simulink model "twoFingerTest2015a"  (R2015a)
settings: Solver=ode45  StartTime=0.0  StopTime=1.0  RelTol=1e-3
settings Model: CovModelRefEnable=off  Creator=Ricardo  LastModifiedBy=Ricardo
settings DataIOCC: SaveFormat=Dataset
settings HardwareCC: ProdBitPerPointer=64  ProdLargestAtomicFloat=Float  ProdIntDivRoundTo=Zero  ProdEndianess=LittleEndian  ProdHWDeviceType=Specified
settings GRTTargetCC: GeneratePreprocessorConditionals=Use local settings

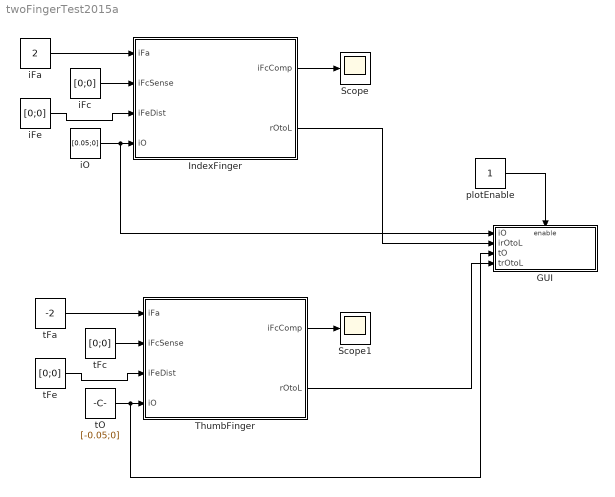
== system twoFingerTest2015a ==
  GUI : Subsystem  TreatAsAtomicUnit=on
  IndexFinger : Subsystem
  Scope : Scope
      settings: TimeRange=auto  MaxDataPoints=5000  SaveToWorkspace=off  SaveName=ScopeData  YMin=-0.27034  YMax=0.08548  SampleTime=-1
  Scope1 : Scope
      settings: TimeRange=auto  MaxDataPoints=5000  SaveToWorkspace=off  YMin=-0.03724  YMax=0.26498  SampleTime=-1
  ThumbFinger : Subsystem
  iFa : Constant  Value=2
  iFc : Constant  Value=[0;0]
  iFe : Constant  Value=[0;0]
  iO : Constant  Value=[0.05;0]
  plotEnable : Constant
  tFa : Constant  Value=-2
  tFc : Constant  Value=[0;0]
  tFe : Constant  Value=[0;0]
  tO : Constant  Value=[-0.05;0]
  wires:
  plotEnable/1 -> GUI/Enable
  IndexFinger/1(iFcComp) -> Scope/1
  iFc/1 -> IndexFinger/2(iFcSense)
  iFe/1 -> IndexFinger/3(iFeDist)
  iO/1 -> GUI/1(iO), IndexFinger/4(iO)
  iFa/1 -> IndexFinger/1(iFa)
  IndexFinger/2(rOtoL) -> GUI/2(irOtoL)
  tFe/1 -> ThumbFinger/3(iFeDist)
  tFa/1 -> ThumbFinger/1(iFa)
  tFc/1 -> ThumbFinger/2(iFcSense)
  tO/1 -> GUI/3(tO), ThumbFinger/4(iO)
  ThumbFinger/1(iFcComp) -> Scope1/1
  ThumbFinger/2(rOtoL) -> GUI/4(trOtoL)

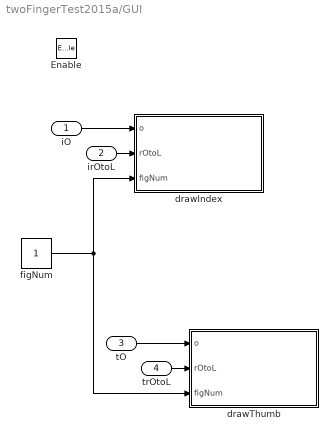
== system twoFingerTest2015a/GUI ==
  iO : Inport
  irOtoL : Inport  Port=2
  tO : Inport  Port=3
  trOtoL : Inport  Port=4
  Enable : EnablePort
  drawIndex : MATLAB Function  TreatAsAtomicUnit=on
      settings: PermitHierarchicalResolution=ParametersOnly
  drawThumb : MATLAB Function  TreatAsAtomicUnit=on
      settings: PermitHierarchicalResolution=ParametersOnly
  figNum : Constant
  wires:
  figNum/1 -> drawThumb/3(figNum), drawIndex/3(figNum)
  tO/1 -> drawThumb/1(o)
  trOtoL/1 -> drawThumb/2(rOtoL)
  irOtoL/1 -> drawIndex/2(rOtoL)
  iO/1 -> drawIndex/1(o)

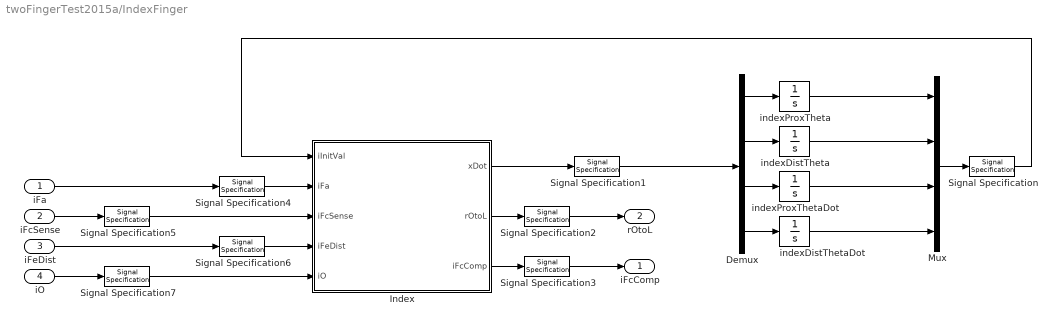
== system twoFingerTest2015a/IndexFinger ==
  iFa : Inport
  iFcSense : Inport  Port=2
  iFeDist : Inport  Port=3
  iO : Inport  Port=4
  Demux : Demux
  Index : MATLAB Function  TreatAsAtomicUnit=on
      settings: PermitHierarchicalResolution=ParametersOnly
  Mux : Mux
  Signal Specification : SignalSpecification  Dimensions=4
  Signal Specification1 : SignalSpecification  Dimensions=4
  Signal Specification2 : SignalSpecification  Dimensions=[2 2]
  Signal Specification{3,5..7} (4 alike) : SignalSpecification  Dimensions=[2 1]
  Signal Specification4 : SignalSpecification  Dimensions=1
  indexDistTheta : Integrator  InitialCondition=pi/3  ContinuousStateAttributes='indexDistTheta'
  indexDistThetaDot : Integrator  ContinuousStateAttributes='indexDistThetaDot'
  indexProxTheta : Integrator  InitialCondition=pi/10  ContinuousStateAttributes='indexProxTheta'
  indexProxThetaDot : Integrator  ContinuousStateAttributes='indexProxThetaDot'
  iFcComp : Outport
  rOtoL : Outport  Port=2
  wires:
  Demux/1 -> indexProxTheta/1
  Demux/2 -> indexDistTheta/1
  Demux/3 -> indexProxThetaDot/1
  Demux/4 -> indexDistThetaDot/1
  indexProxTheta/1 -> Mux/1
  indexDistTheta/1 -> Mux/2
  indexProxThetaDot/1 -> Mux/3
  indexDistThetaDot/1 -> Mux/4
  Index/1(xDot) -> Signal Specification1/1
  Mux/1 -> Signal Specification/1
  Index/2(rOtoL) -> Signal Specification2/1
  Signal Specification/1 -> Index/1(iInitVal)
  Signal Specification1/1 -> Demux/1
  iFa/1 -> Signal Specification4/1
  iFcSense/1 -> Signal Specification5/1
  iFeDist/1 -> Signal Specification6/1
  iO/1 -> Signal Specification7/1
  Signal Specification2/1 -> rOtoL/1
  Signal Specification3/1 -> iFcComp/1
  Index/3(iFcComp) -> Signal Specification3/1
  Signal Specification4/1 -> Index/2(iFa)
  Signal Specification5/1 -> Index/3(iFcSense)
  Signal Specification6/1 -> Index/4(iFeDist)
  Signal Specification7/1 -> Index/5(iO)

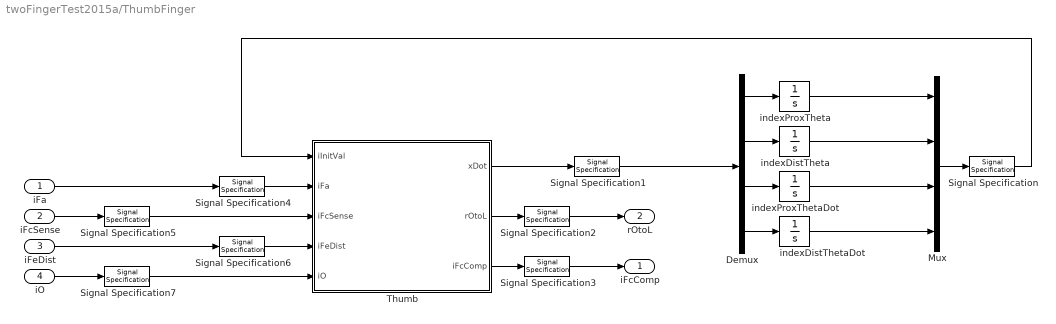
== system twoFingerTest2015a/ThumbFinger ==
  iFa : Inport
  iFcSense : Inport  Port=2
  iFeDist : Inport  Port=3
  iO : Inport  Port=4
  Demux : Demux
  Mux : Mux
  Signal Specification : SignalSpecification  Dimensions=4
  Signal Specification1 : SignalSpecification  Dimensions=4
  Signal Specification2 : SignalSpecification  Dimensions=[2 2]
  Signal Specification{3,5..7} (4 alike) : SignalSpecification  Dimensions=[2 1]
  Signal Specification4 : SignalSpecification  Dimensions=1
  Thumb : MATLAB Function  TreatAsAtomicUnit=on
      settings: PermitHierarchicalResolution=ParametersOnly
  indexDistTheta : Integrator  InitialCondition=-pi/3  ContinuousStateAttributes='indexDistTheta'
  indexDistThetaDot : Integrator  ContinuousStateAttributes='indexDistThetaDot'
  indexProxTheta : Integrator  InitialCondition=pi-pi/10  ContinuousStateAttributes='indexProxTheta'
  indexProxThetaDot : Integrator  ContinuousStateAttributes='indexProxThetaDot'
  iFcComp : Outport
  rOtoL : Outport  Port=2
  wires:
  Demux/1 -> indexProxTheta/1
  Demux/2 -> indexDistTheta/1
  Demux/3 -> indexProxThetaDot/1
  Demux/4 -> indexDistThetaDot/1
  indexProxTheta/1 -> Mux/1
  indexDistTheta/1 -> Mux/2
  indexProxThetaDot/1 -> Mux/3
  indexDistThetaDot/1 -> Mux/4
  Thumb/1(xDot) -> Signal Specification1/1
  Mux/1 -> Signal Specification/1
  Thumb/2(rOtoL) -> Signal Specification2/1
  Signal Specification/1 -> Thumb/1(iInitVal)
  Signal Specification1/1 -> Demux/1
  iFa/1 -> Signal Specification4/1
  iFcSense/1 -> Signal Specification5/1
  iFeDist/1 -> Signal Specification6/1
  iO/1 -> Signal Specification7/1
  Signal Specification2/1 -> rOtoL/1
  Signal Specification3/1 -> iFcComp/1
  Thumb/3(iFcComp) -> Signal Specification3/1
  Signal Specification4/1 -> Thumb/2(iFa)
  Signal Specification5/1 -> Thumb/3(iFcSense)
  Signal Specification6/1 -> Thumb/4(iFeDist)
  Signal Specification7/1 -> Thumb/5(iO)

== matlab function twoFingerTest2015a/GUI/drawThumb ==
  data: o input; rOtoL input; figNum input
% Plots finger to the default figure. Handled in Simulink.
% Author: Ricardo Garcia Rosas
% Change log:
%%%%%%%%%%%%|%%%%%%%%%%%|%%%%%%%%%%%%%%%%%%%%%%%%%%%%%%%%%%%%%%%%%%%|
% Date      |   Author  | Notes                                     |
% 16/03/23  |   RGR     | Added more comments.                      |
function drawFinger(o,rOtoL,figNum)
    % Plots the finger to the default figure. Handled in Simulink.
    % @param o finger origin position [x,y] (m).
    % @param rOtoL finger vector from its origin to its link
    % ends.
    % @param figNum the figure number for the plot.

    % Call figure
    figure(figNum);
    hold on;
    % Draw Proximal components
    plot([o(1) rOtoL(1,1)],[o(2) rOtoL(2,1)],'LineWidth',8,'Color', 'k');
    plot(o(1),o(2),'ko','MarkerSize',18);
    % Draw Distal components
    plot([rOtoL(1,1) rOtoL(1,2)],[rOtoL(2,1) rOtoL(2,2)],'LineWidth',8,'Color', 'k');
    plot(rOtoL(1,1),rOtoL(2,1),'ko','MarkerSize',18);
    % Draw fingertip
    plot(rOtoL(1,2),rOtoL(2,2),'ko','MarkerSize',8);
    hold off;
    axis([-0.2 0.2 -0.05 0.2]);
end

== matlab function twoFingerTest2015a/IndexFinger/Index ==
  data: iInitVal input; xDot output; iFa input; iFcSense input; iFeDist input; iO input; rOtoL output; iFcComp output
% Finger Simulink function.
% Represents an underactuated cable driven finger.
% The finger is composed of two phalanges driven by a tendon-pulley
% mechanism. This has methods for calculating the kinematics and
% dynamics of the system.
% Author: Ricardo Garcia Rosas
% Change log:
%%%%%%%%%%%%|%%%%%%%%%%%|%%%%%%%%%%%%%%%%%%%%%%%%%%%%%%%%%%%%%%%%%%%|
% Date      |   Author  | Notes                                     |
% 16/03/23  |   RGR     | Added more comments.                      |
% 16/03/24  |   RGR     | Compute fc and transform to [x,y].        |
% 16/04/06  |   RGR     | Removed force class, using only magnitude.|
% 16/04/09  |   RGR     | Removed classes and opted for functions.  |

function [ xDot, rOtoL, iFcComp ] = Finger( iInitVal,iFa,iFcSense,iFeDist,iO )

    % Set initial condition:
    theta = [iInitVal(1); iInitVal(2)];
    thetaDot = [iInitVal(3); iInitVal(4)];
    % Transform forces:
    % Contact force
    fcTN = rotMat(theta(1,1)+theta(2,1))'*iFcSense;
    fcD = fcTN(2,1);
    % Disturbance force
    feTN = rotMat(theta(1,1)+theta(2,1))'*iFeDist;
    feD = feTN(2,1);
    % Set model variables:
    kP = -0.043;
    kD = -0.185;
    dP = -0.01;
    dD = -0.01;
    lP = 0.1;
    lD = 0.1;
    rP = 0.02;
    rD = 0.012;
    aP = 0.1;
    aD = 0.1;
    bP = 0.05;
    bD = 0.05;
    mP = 0.02;
    mD = 0.02;
    theta0 = [pi/10;pi/3];
    IP = mP*(lP^2)/3;
    ID = mD*(lD^2)/12;
    % Set matrices
    K = [kP 0;
         0 kD];
    D = [dP 0;
         0 dD];
    Ja = [rP rD];
    Jc = [aP, 0;
          aD+lP*cos(theta(2,1)),aD];
    Je = [bP, 0;
          bD+lP*cos(theta(2,1)),bD]; 

    % Forward kinematics to link ends and centre of gravity.
    % rOtoL vector from finger origin to link end, one 2D
    % vector for each link.
    % rOtoG vector from finger origin to link center of
    % gravity, one 2D vector for each link.
    rOtoL = zeros(2,2);
    rOtoG = zeros(2,2);
    rOtoL(:,1) = iO + rotMat(theta(1,1))*[lP;0];
    rOtoG(:,1) = iO + rotMat(theta(1,1))*[lP/2;0];
    rOtoL(:,2) = rOtoL(:,2-1) + rotMat(theta(1,1)+theta(2,1))*[lD;0];
    rOtoG(:,2) = rOtoG(:,2-1) + rotMat(theta(1,1)+theta(2,1))*[lD/2;0];
    
    % Dyniamics
    % Compute matrix parameters.
    alpha = IP + ID + (mP*(lP/2)^2) + mD*(lP^2+(lD/2)^2);
    beta = mD*lP*(lD/2);
    delta = ID+mD*(lD/2)^2;
    % Intertia matrix (M)
    M = [alpha+2*beta*cos(theta(2,1)) delta+beta*cos(theta(2,1));
         delta+beta*cos(theta(2,1)) delta];
    % Coriolis and Centrifugal matrix (C)
    C = [-beta*sin(theta(2,1))*thetaDot(2,1) ...
         -beta*sin(theta(2,1))*(thetaDot(1,1)+thetaDot(2,1));
         beta*sin(theta(2,1))*thetaDot(1,1) 0];
    % Torques
    springTau = K*(theta-theta0);
    damperTau = D*thetaDot;
    contactTau = Jc'*[0; fcD];
    distTau = Je'*[0; feD];
    actTau = Ja'*iFa;
    % Compute angular acceleration
    thetaDotDot = inv(M)*(-C*thetaDot + springTau + damperTau + contactTau + distTau + actTau);
    xDot = [thetaDot; thetaDotDot];
    % Compute applied contact force give a static condition. (Kinetostatic)
    % Compute forces normal to proximal and distal links.
    fcComp = (inv(Jc')*-(springTau+damperTau+distTau+actTau));
    % Distal normal and tangential (0, no tangential force due to
    % actuation) forces and transform to [x,y] coordinate.
    iFcComp = -rotMat(theta(1,1)+theta(2,1))*[0;fcComp(2)];
end
        function rot = rotMat(theta)
            % 2D Z-Rotation matrix on theta.
            % @param theta the angle
            % @return rot the rotation matrix as a 2x2 matrix.
            rot = [cos(theta) -sin(theta);
                   sin(theta) cos(theta)];
        end

== matlab function twoFingerTest2015a/ThumbFinger/Thumb ==
  data: iInitVal input; xDot output; iFa input; iFcSense input; iFeDist input; iO input; rOtoL output; iFcComp output
% Finger Simulink function.
% Represents an underactuated cable driven finger.
% The finger is composed of two phalanges driven by a tendon-pulley
% mechanism. This has methods for calculating the kinematics and
% dynamics of the system.
% Author: Ricardo Garcia Rosas
% Change log:
%%%%%%%%%%%%|%%%%%%%%%%%|%%%%%%%%%%%%%%%%%%%%%%%%%%%%%%%%%%%%%%%%%%%|
% Date      |   Author  | Notes                                     |
% 16/03/23  |   RGR     | Added more comments.                      |
% 16/03/24  |   RGR     | Compute fc and transform to [x,y].        |
% 16/04/06  |   RGR     | Removed force class, using only magnitude.|
% 16/04/09  |   RGR     | Removed classes and opted for functions.  |

function [ xDot, rOtoL, iFcComp ] = Finger( iInitVal,iFa,iFcSense,iFeDist,iO )

    % Set initial condition:
    theta = [iInitVal(1); iInitVal(2)];
    thetaDot = [iInitVal(3); iInitVal(4)];
    % Transform forces:
    % Contact force
    fcTN = rotMat(theta(1,1)+theta(2,1))'*iFcSense;
    fcD = fcTN(2,1);
    % Disturbance force
    feTN = rotMat(theta(1,1)+theta(2,1))'*iFeDist;
    feD = feTN(2,1);
    % Set model variables:
    kP = -0.043;
    kD = -0.185;
    dP = -0.01;
    dD = -0.01;
    lP = 0.1;
    lD = 0.1;
    rP = 0.02;
    rD = 0.012;
    aP = 0.1;
    aD = 0.1;
    bP = 0.05;
    bD = 0.05;
    mP = 0.02;
    mD = 0.02;
    theta0 = [pi-pi/10;-pi/3];
    IP = mP*(lP^2)/3;
    ID = mD*(lD^2)/12;
    % Set matrices
    K = [kP 0;
         0 kD];
    D = [dP 0;
         0 dD];
    Ja = [rP rD];
    Jc = [aP, 0;
          aD+lP*cos(theta(2,1)),aD];
    Je = [bP, 0;
          bD+lP*cos(theta(2,1)),bD]; 

    % Forward kinematics to link ends and centre of gravity.
    % rOtoL vector from finger origin to link end, one 2D
    % vector for each link.
    % rOtoG vector from finger origin to link center of
    % gravity, one 2D vector for each link.
    rOtoL = zeros(2,2);
    rOtoG = zeros(2,2);
    rOtoL(:,1) = iO + rotMat(theta(1,1))*[lP;0];
    rOtoG(:,1) = iO + rotMat(theta(1,1))*[lP/2;0];
    rOtoL(:,2) = rOtoL(:,2-1) + rotMat(theta(1,1)+theta(2,1))*[lD;0];
    rOtoG(:,2) = rOtoG(:,2-1) + rotMat(theta(1,1)+theta(2,1))*[lD/2;0];
    
    % Dyniamics
    % Compute matrix parameters.
    alpha = IP + ID + (mP*(lP/2)^2) + mD*(lP^2+(lD/2)^2);
    beta = mD*lP*(lD/2);
    delta = ID+mD*(lD/2)^2;
    % Intertia matrix (M)
    M = [alpha+2*beta*cos(theta(2,1)) delta+beta*cos(theta(2,1));
         delta+beta*cos(theta(2,1)) delta];
    % Coriolis and Centrifugal matrix (C)
    C = [-beta*sin(theta(2,1))*thetaDot(2,1) ...
         -beta*sin(theta(2,1))*(thetaDot(1,1)+thetaDot(2,1));
         beta*sin(theta(2,1))*thetaDot(1,1) 0];
    % Torques
    springTau = K*(theta-theta0);
    damperTau = D*thetaDot;
    contactTau = Jc'*[0; fcD];
    distTau = Je'*[0; feD];
    actTau = Ja'*iFa;
    % Compute angular acceleration
    thetaDotDot = inv(M)*(-C*thetaDot + springTau + damperTau + contactTau + distTau + actTau);
    xDot = [thetaDot; thetaDotDot];
    % Compute applied contact force give a static condition. (Kinetostatic)
    % Compute forces normal to proximal and distal links.
    fcComp = (inv(Jc')*-(springTau+damperTau+distTau+actTau));
    % Distal normal and tangential (0, no tangential force due to
    % actuation) forces and transform to [x,y] coordinate.
    iFcComp = -rotMat(theta(1,1)+theta(2,1))*[0;fcComp(2)];
end
        function rot = rotMat(theta)
            % 2D Z-Rotation matrix on theta.
            % @param theta the angle
            % @return rot the rotation matrix as a 2x2 matrix.
            rot = [cos(theta) -sin(theta);
                   sin(theta) cos(theta)];
        end

== matlab function twoFingerTest2015a/GUI/drawIndex ==
  data: o input; rOtoL input; figNum input
% Plots finger to the default figure. Handled in Simulink.
% Author: Ricardo Garcia Rosas
% Change log:
%%%%%%%%%%%%|%%%%%%%%%%%|%%%%%%%%%%%%%%%%%%%%%%%%%%%%%%%%%%%%%%%%%%%|
% Date      |   Author  | Notes                                     |
% 16/03/23  |   RGR     | Added more comments.                      |
function drawFinger(o,rOtoL,figNum)
    % Plots the finger to the default figure. Handled in Simulink.
    % @param o finger origin position [x,y] (m).
    % @param rOtoL finger vector from its origin to its link
    % ends.
    % @param figNum the figure number for the plot.

    % Call figure
    figure(figNum);
    clf;
    hold on;
    % Draw Proximal components
    plot([o(1) rOtoL(1,1)],[o(2) rOtoL(2,1)],'LineWidth',8,'Color', 'k');
    plot(o(1),o(2),'ko','MarkerSize',18);
    % Draw Distal components
    plot([rOtoL(1,1) rOtoL(1,2)],[rOtoL(2,1) rOtoL(2,2)],'LineWidth',8,'Color', 'k');
    plot(rOtoL(1,1),rOtoL(2,1),'ko','MarkerSize',18);
    % Draw fingertip
    plot(rOtoL(1,2),rOtoL(2,2),'ko','MarkerSize',8);
    hold off;
    axis([-0.2 0.2 -0.05 0.2]);
end
